simulink model "sampleModel333"  (R2021b)
settings: Solver=VariableStepAuto  StartTime=0.0  StopTime=10.0  RelTol=1e-3
libraries: simulink x4
settings Model: Creator=user  LastModifiedBy=user

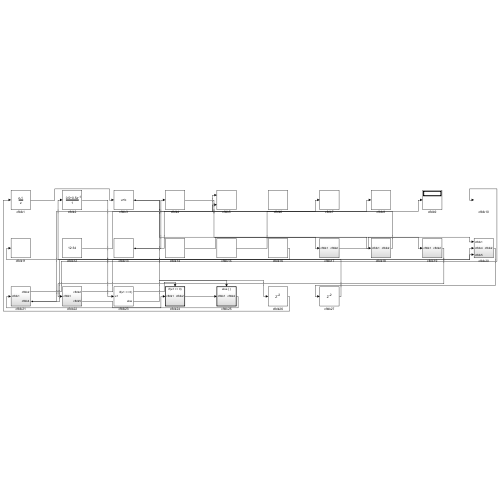
[thumbnail: Simulink's stored preview of the top-level diagram]
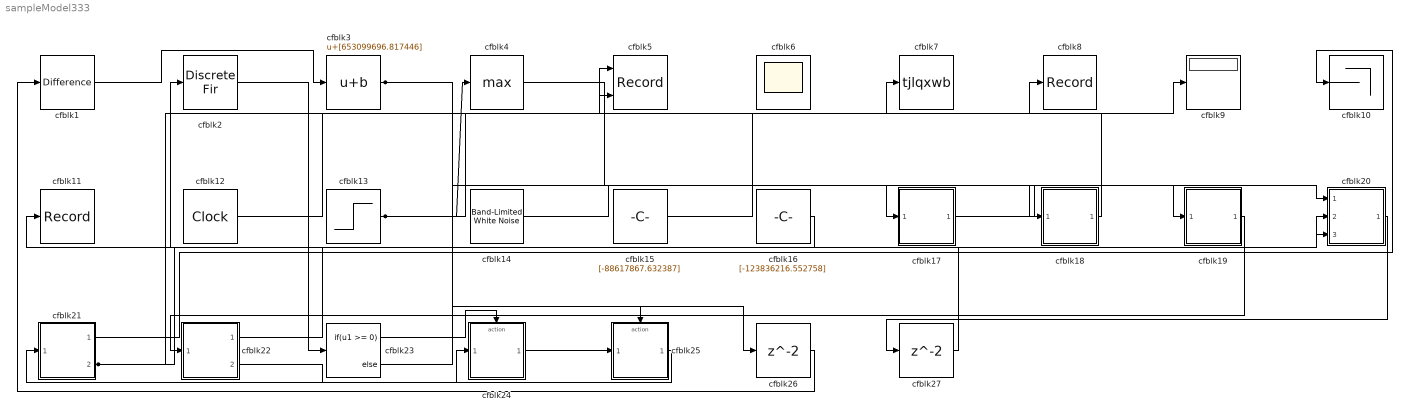
== system sampleModel333 ==
  cfblk1 : simulink/Discrete/Difference  ICPrevInput=0.0  OutMin=[]  OutMax=[]  OutDataTypeStr=Inherit: Inherit via back propagation  OutDataType=fixdt(1, 16)  OutScaling=2^-10  DoSatur=off
  cfblk10 : Terminator
  cfblk11 : Record  FileSettingsInternal="{\"entries\":[{\"content\":{\"excelSettings\":{\"content\":{},\"type\":\"Streamout.ExcelSettings\"}},\"type\":\"Streamout.FileSettingStorage\",\"uuid\":\"5ce30b26-9ff3-4ded-a506-6321216ec595\"}],\"packageUris\":[\"http://schema.mathworks.com/mf0/streamout_blocks/R2020a\"],\"version\":\"1.0\"}"  SignalsInternal="{\"entries\":[{\"content\":{\"signals\":[{\"content\":{\"blockPath\":[\"sampleModel333/cfblk11\"],\"channel\":[],\"dimensions\":[1],\"domain\":\"sampleModel333/cfblk11\",\"lineColor\":\"#4dbeee\",\"plots\":[1],\"port\":1,\"sid\":[\"\"],\"signalID\":14047,\"signalName\":\"cfblk16\"},\"type\":\"RecordBlkView.Signal\",\"uuid\":\"64764909-9324-44b7-839a-83af6aa2e04c\"}]},\"type\":\"RecordBlkView.InputSignals\",\"uuid\":\"01ae6be7-dfd3-4efb-a269-0df1d3eb45b1\"}],\"packageUris\":[\"http://schema.mathworks.com/mf0/streamout_blocks/R2020a\"],\"version\":\"1.0\"}"  VisualizationBindings="{\"sparklinesplugin\":{\"info\":[{\"bindingParametersList\":[],\"subplotID\":1}]}}"
  cfblk12 : DigitalClock
  cfblk13 : Step  Time=[22.000000]  Before=[899629516.605013]  After=[332212343.267808]  SampleTime=0
  cfblk14 : simulink/Sources/Band-Limited White Noise  Cov=[4632986096.393378]  Ts=0.1  seed=[3360259371.000000]
  cfblk15 : Constant  Value=[-88617867.632387]  SampleTime=1
  cfblk16 : Constant  Value=[-123836216.552758]  SampleTime=1
  cfblk17 : Subsystem
  cfblk18 : Subsystem
  cfblk19 : Subsystem
  cfblk2 : DiscreteFir  SampleTime=1
  cfblk20 : Subsystem
  cfblk21 : Subsystem
  cfblk22 : Subsystem
  cfblk23 : If  IfExpression=u1 >= 0  SampleTime=1
  cfblk24 : Subsystem  TreatAsAtomicUnit=on
  cfblk25 : Subsystem  TreatAsAtomicUnit=on
  cfblk26 : Delay  SampleTime=1
  cfblk27 : Delay  SampleTime=1
  cfblk3 : Bias  Bias=[653099696.817446]
  cfblk4 : MinMax  Function=max
  cfblk5 : Record  FileSettingsInternal="{\"entries\":[{\"content\":{\"excelSettings\":{\"content\":{},\"type\":\"Streamout.ExcelSettings\"}},\"type\":\"Streamout.FileSettingStorage\",\"uuid\":\"4d4139e4-2404-4219-b25a-6d2be678a3f8\"}],\"packageUris\":[\"http://schema.mathworks.com/mf0/streamout_blocks/R2020a\"],\"version\":\"1.0\"}"  Layout=[1 1]  SignalsInternal="{\"entries\":[{\"content\":{\"signals\":[{\"content\":{\"blockPath\":[\"sampleModel333/cfblk5\"],\"channel\":[],\"dimensions\":[1],\"domain\":\"sampleModel333/cfblk5\",\"lineColor\":\"#a2142f\",\"plots\":[1],\"port\":1,\"sid\":[\"\"],\"signalID\":14039,\"signalName\":\"cfblk18\"},\"type\":\"RecordBlkView.Signal\",\"uuid\":\"cc00fe8a-76cc-4009-8e86-165c892498ed\"},{\"content\":{\"blockPath\":[\"sampleModel333/cfblk5\"],\"channel\":[],\"dimensions\":[1],\"domain\":\"sampleModel333/cfblk5\",\"lineColor\":\"#139fff\",\"plots\":[1],\"port\":2,\"sid\":[\"\"],\"signalID\":14043,\"signalName\":\"cfblk21:2\"},\"type\":\"RecordBlkView.Signal\",\"uuid\":\"9ae7eb75-a026-46ed-9194-37e2bab66e94\"}]},\"type\":\"RecordBlkView.InputSignals\",\"uuid\":\"e42e9141-39d8-4116-8937-4ac3598ae7a9\"}],\"packageUris\":[\"http://schema.mathworks.com/mf0/streamout_blocks/R2020a\"],\"version\":\"1.0\"}"  VisualizationBindings="{\"xyplotplugin\":{\"info\":[{\"series\":[{\"bindingParametersList\":[{\"parameter\":\"X-Axis\",\"signalID\":14039,\"signalName\":\"cfblk18\"},{\"parameter\":\"Y-Axis\",\"signalID\":14043,\"signalName\":\"cfblk21:2\"}],\"seriesID\":23874}],\"subplotID\":1}]}}"  CompatibilityTag=XY
  cfblk6 : Scope
      settings: Floating=on
  cfblk7 : ToWorkspace  VariableName=tjlqxwb  SaveFormat=Timeseries  SampleTime=-1
  cfblk8 : Record  FileSettingsInternal="{\"entries\":[{\"content\":{\"excelSettings\":{\"content\":{},\"type\":\"Streamout.ExcelSettings\"}},\"type\":\"Streamout.FileSettingStorage\",\"uuid\":\"3154be89-9f2a-443c-9c67-711933af3d73\"}],\"packageUris\":[\"http://schema.mathworks.com/mf0/streamout_blocks/R2020a\"],\"version\":\"1.0\"}"  SignalsInternal="{\"entries\":[{\"content\":{\"signals\":[{\"content\":{\"blockPath\":[\"sampleModel333/cfblk8\"],\"channel\":[],\"dimensions\":[1],\"domain\":\"sampleModel333/cfblk8\",\"lineColor\":\"#a2142f\",\"plots\":[1],\"port\":1,\"sid\":[\"\"],\"signalID\":14051,\"signalName\":\"cfblk12\"},\"type\":\"RecordBlkView.Signal\",\"uuid\":\"b25434d1-4f56-473c-ba65-4acbd035b84e\"}]},\"type\":\"RecordBlkView.InputSignals\",\"uuid\":\"c895d658-c348-4248-994b-9a985203ef43\"}],\"packageUris\":[\"http://schema.mathworks.com/mf0/streamout_blocks/R2020a\"],\"version\":\"1.0\"}"  VisualizationBindings="{\"sparklinesplugin\":{\"info\":[{\"bindingParametersList\":[],\"subplotID\":1}]}}"
  cfblk9 : Display
  wires:
  cfblk13/1 -> cfblk4/1, cfblk7/1
  cfblk1/1 -> cfblk3/1
  cfblk25/1(cfblk2) -> cfblk21/1(cfblk1)
  cfblk3/1 -> cfblk18/1(cfblk1), cfblk26/1
  cfblk24/1(cfblk2) -> cfblk25/1(cfblk1)
  cfblk4/1 -> cfblk17/1(cfblk1)
  cfblk16/1 -> cfblk11/1
  cfblk21/1(cfblk2) -> cfblk10/1
  cfblk17/1(cfblk2) -> cfblk19/1(cfblk1)
  cfblk14/1 -> cfblk20/1(cfblk1)
  cfblk18/1(cfblk2) -> cfblk5/1
  cfblk21/2(cfblk4) -> cfblk20/2(cfblk4), cfblk5/2
  cfblk12/1 -> cfblk8/1
  cfblk15/1 -> cfblk9/1
  cfblk19/1(cfblk2) -> cfblk22/1(cfblk1)
  cfblk2/1 -> cfblk23/1
  cfblk22/1(cfblk2) -> cfblk20/3(cfblk5)
  cfblk22/2(cfblk5) -> cfblk24/1(cfblk1)
  cfblk23/1 -> cfblk24/Action
  cfblk23/2 -> cfblk25/Action
  cfblk26/1 -> cfblk1/1
  cfblk20/1(cfblk2) -> cfblk27/1
  cfblk27/1 -> cfblk2/1

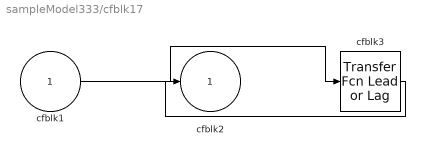
== system sampleModel333/cfblk17 ==
  cfblk1 : Inport
  cfblk3 : simulink/Discrete/Transfer Fcn Lead or Lag  PoleZ=0.95  ZeroZ=0.75  ICPrevOutput=0.0  ICPrevInput=0.0  DoSatur=off
      settings: SourceProductBaseCode=SL
  cfblk2 : Outport
  wires:
  cfblk1/1 -> cfblk3/1
  cfblk3/1 -> cfblk2/1

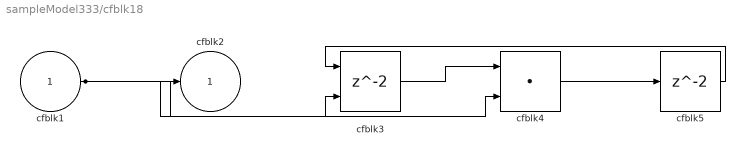
== system sampleModel333/cfblk18 ==
  cfblk1 : Inport
  cfblk3 : Delay  ShowEnablePort=on  SampleTime=1
      settings: InputPortMap=u0,e6
  cfblk4 : DotProduct  InputSameDT=on  OutDataTypeStr=Inherit: Inherit via internal rule
  cfblk5 : Delay  SampleTime=1
  cfblk2 : Outport
  wires:
  cfblk1/1 -> cfblk3/2, cfblk2/1, cfblk4/2
  cfblk3/1 -> cfblk4/1
  cfblk4/1 -> cfblk5/1
  cfblk5/1 -> cfblk3/1

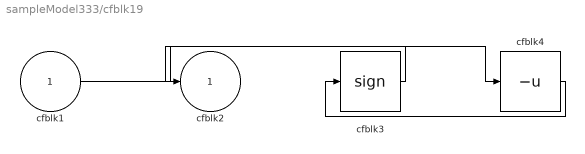
== system sampleModel333/cfblk19 ==
  cfblk1 : Inport
  cfblk3 : Signum
  cfblk4 : UnaryMinus
  cfblk2 : Outport
  wires:
  cfblk1/1 -> cfblk4/1
  cfblk4/1 -> cfblk3/1
  cfblk3/1 -> cfblk2/1

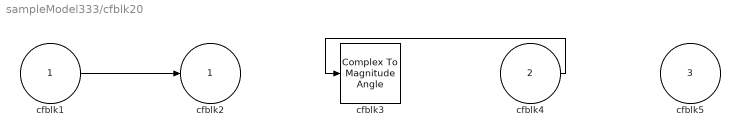
== system sampleModel333/cfblk20 ==
  cfblk1 : Inport
  cfblk4 : Inport  Port=2
  cfblk5 : Inport  Port=3
  cfblk3 : ComplexToMagnitudeAngle
  cfblk2 : Outport
  wires:
  cfblk1/1 -> cfblk2/1
  cfblk4/1 -> cfblk3/1

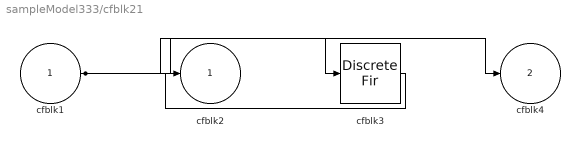
== system sampleModel333/cfblk21 ==
  cfblk1 : Inport
  cfblk3 : DiscreteFir  SampleTime=1
  cfblk2 : Outport
  cfblk4 : Outport  Port=2
  wires:
  cfblk1/1 -> cfblk4/1, cfblk3/1
  cfblk3/1 -> cfblk2/1

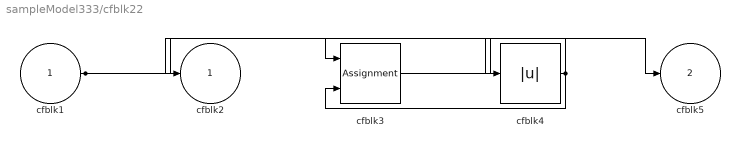
== system sampleModel333/cfblk22 ==
  cfblk1 : Inport
  cfblk3 : Assignment  DiagnosticForDimensions=Warning  IndexOptions=Index vector (dialog)  Indices=1  OutputSizes=1
  cfblk4 : Abs
  cfblk2 : Outport
  cfblk5 : Outport  Port=2
  wires:
  cfblk1/1 -> cfblk3/1, cfblk4/1
  cfblk4/1 -> cfblk3/2, cfblk2/1
  cfblk3/1 -> cfblk5/1

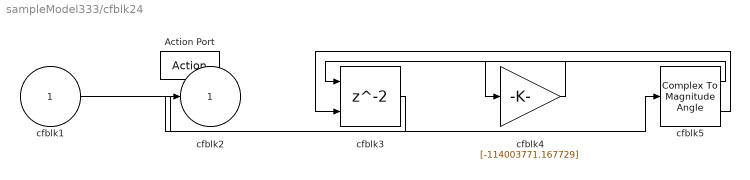
== system sampleModel333/cfblk24 ==
  cfblk1 : Inport
  Action Port : ActionPort  ActionPortLabel=if(u1 >= 0)
  cfblk3 : Delay  ShowEnablePort=on
      settings: InputPortMap=u0,e6
  cfblk4 : Gain  Gain=[-114003771.167729]
  cfblk5 : ComplexToMagnitudeAngle
  cfblk2 : Outport
  wires:
  cfblk4/1 -> cfblk3/1
  cfblk1/1 -> cfblk5/1
  cfblk5/1 -> cfblk4/1
  cfblk5/2 -> cfblk3/2
  cfblk3/1 -> cfblk2/1

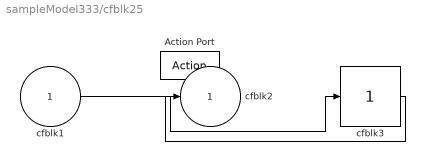
== system sampleModel333/cfblk25 ==
  cfblk1 : Inport
  Action Port : ActionPort  ActionPortLabel=else
  cfblk3 : simulink/Math Operations/Slider Gain  gain=1  low=0  high=2
  cfblk2 : Outport
  wires:
  cfblk1/1 -> cfblk3/1
  cfblk3/1 -> cfblk2/1
